simulink model "controladorNovo2015"  (R2018a)
settings: Solver=VariableStepAuto  StartTime=0.0  StopTime=Tsimu  FixedStep=h  RelTol=1e-3
values from neighbouring files (symbols this model uses):
  G = [1; 1]    [init.m]
  h = 0.01    [init.m]
  P0 = eye(2)*1e-4*100    [init.m]
  Qn = 0.01    [init.m]
  R = 0.01    [init.m]
  x0 = x0barra + epsilon    [init.m]
  x0hat = x0barra    [init.m]
undefined symbols (not defined in the file or in its folder): C, Cd, gama, H, phi, Tsimu
libraries: dspinverses x2, dspsrcs4 x1
settings Model: Creator=Raposo  LastModifiedBy=Raposo
settings OptimizationCC: LifeSpan=inf
settings DebuggingCC: AllowSymbolicDim=off  SFExecutionAtInitializationDiag=none
settings HardwareCC: ProdBitPerSizeT=32  ProdBitPerPtrDiffT=32  ProdWordSize=32  ProdHWDeviceType=Specified
settings CodeAppCC: StateflowObjectComments=on

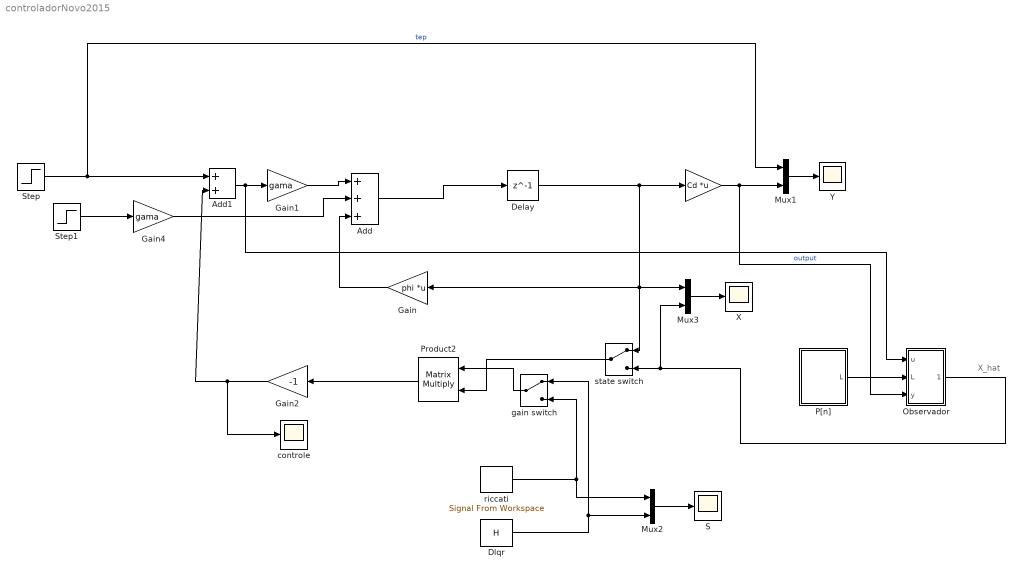
== system controladorNovo2015 ==
  note: X_hat
  " " : Gain  Gain=Cd  Multiplication=Matrix(K*u)
  Add : Sum  Inputs=+++
  Add1 : Sum
  Delay : Delay  DelayLength=1  InitialCondition=x0  SampleTime=h
  Dlqr : Constant  Value=H  VectorParams1D=off
  Gain : Gain  Gain=phi  Multiplication=Matrix(K*u)
  Gain1 : Gain  Gain=gama
  Gain2 : Gain  Gain=-1
  Gain4 : Gain  Gain=gama
  Mux1 : Mux  Inputs=2
  Mux2 : Mux  Inputs=2
  Mux3 : Mux  Inputs=2
  "Observador " : Subsystem
  P[n] : Subsystem
  Product2 : Product  Multiplication=Matrix(*)
  S : Scope
  Step : Step  Time=Tsimu/2  SampleTime=h
  Step1 : Step  Time=10  After=0  SampleTime=1
  X : Scope
  Y : Scope
  controle : Scope
  gain switch : ManualSwitch
  riccati : dspsrcs4/Signal From Workspace  X=lx'  Ts=1  nsamps=1  OutputAfterFinalValue=Setting to zero  ignoreOrWarnInputAndFrameLengths=off  OutputFrames=on
  state switch : ManualSwitch
  wires:
  Gain/1 -> Add/3
  Delay/1 -> Mux3/1, state switch/1, Gain/1, " "/1
  riccati/1 -> Mux2/1, gain switch/2
  Step/1 -> Mux1/1, Add1/1  "tep"
  Mux1/1 -> Y/1
  " "/1 -> "Observador "/3("y "), Mux1/2  "output"
  Mux2/1 -> S/1
  Add1/1 -> "Observador "/1(u), Gain1/1
  Gain1/1 -> Add/1
  Add/1 -> Delay/1
  Product2/1 -> Gain2/1
  Gain2/1 -> controle/1, Add1/2
  Dlqr/1 -> Mux2/2, gain switch/1
  gain switch/1 -> Product2/1
  P[n]/1(L) -> "Observador "/2(L)
  state switch/1 -> Product2/2
  "Observador "/1(Out1) -> Mux3/2, state switch/2
  Mux3/1 -> X/1
  Gain4/1 -> Add/2
  Step1/1 -> Gain4/1

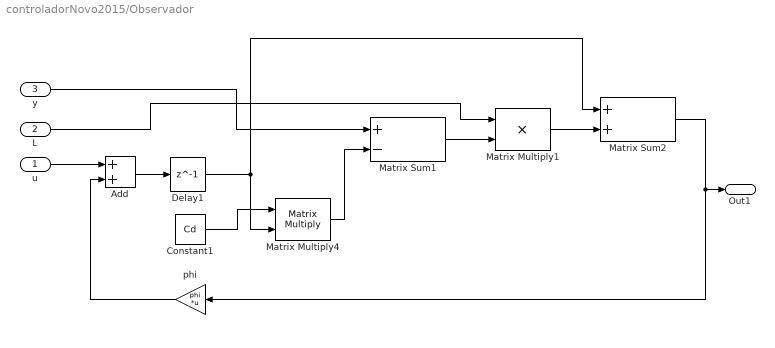
== system controladorNovo2015/Observador  ==
  u : Inport
  L : Inport  Port=2
  "y " : Inport  Port=3
  Add : Sum
  Constant1 : Constant  Value=Cd  VectorParams1D=off
  Delay1 : Delay  DelayLength=1  InitialCondition=x0hat
  Matrix Sum1 : Sum  Inputs=+-
  Matrix Sum2 : Sum
  Matrix Multiply1 : Product  Inputs=**
  Matrix Multiply4 : Product  Inputs=**  Multiplication=Matrix(*)
  phi : Gain  Gain=phi  Multiplication=Matrix(K*u)
  Out1 : Outport
  wires:
  phi/1 -> Add/2
  u/1 -> Add/1
  Add/1 -> Delay1/1
  Matrix Sum2/1 -> Out1/1, phi/1
  "y "/1 -> Matrix Sum1/1
  Delay1/1 -> Matrix Multiply4/2, Matrix Sum2/1
  L/1 -> Matrix Multiply1/1
  Constant1/1 -> Matrix Multiply4/1
  Matrix Multiply4/1 -> Matrix Sum1/2
  Matrix Sum1/1 -> Matrix Multiply1/2
  Matrix Multiply1/1 -> Matrix Sum2/2

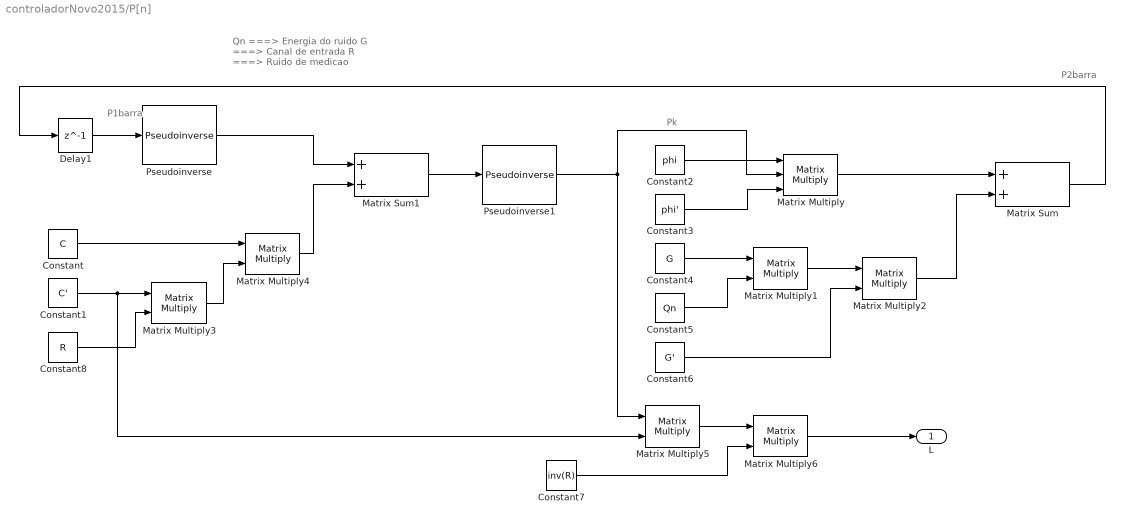
== system controladorNovo2015/P[n] ==
  note: Pk
  note: Qn ===> Energia do ruido
      | G   ===> Canal de entrada
      | R   ===> Ruido de medicao
  note: P2barra
  note: P1barra
  Constant : Constant  Value=C  VectorParams1D=off
  Constant1 : Constant  Value=C'  VectorParams1D=off
  Constant2 : Constant  Value=phi  VectorParams1D=off
  Constant3 : Constant  Value=phi'  VectorParams1D=off
  Constant4 : Constant  Value=G  VectorParams1D=off
  Constant5 : Constant  Value=Qn  VectorParams1D=off
  Constant6 : Constant  Value=G'  VectorParams1D=off
  Constant7 : Constant  Value=inv(R)  VectorParams1D=off
  Constant8 : Constant  Value=R  VectorParams1D=off
  Delay1 : Delay  DelayLength=1  InitialCondition=P0
  Matrix Sum : Sum
  Matrix Sum1 : Sum
  Matrix Multiply : Product  Inputs=***  Multiplication=Matrix(*)
  Matrix Multiply{1..6} (6 alike) : Product  Inputs=**  Multiplication=Matrix(*)
  Pseudoinverse : dspinverses/Pseudoinverse  wanterr=off  SimulateUsing=Interpreted execution
      settings: SourceProductName=DSP System Toolbox  SourceProductBaseCode=DS
  Pseudoinverse1 : dspinverses/Pseudoinverse  wanterr=off  SimulateUsing=Interpreted execution
      settings: SourceProductName=DSP System Toolbox  SourceProductBaseCode=DS
  L : Outport
  wires:
  Pseudoinverse1/1 -> Matrix Multiply5/1, Matrix Multiply/2
  Matrix Sum/1 -> Delay1/1
  Matrix Multiply6/1 -> L/1
  Delay1/1 -> Pseudoinverse/1
  Constant/1 -> Matrix Multiply4/1
  Constant1/1 -> Matrix Multiply5/2, Matrix Multiply3/1
  Constant2/1 -> Matrix Multiply/1
  Constant3/1 -> Matrix Multiply/3
  Constant4/1 -> Matrix Multiply1/1
  Constant5/1 -> Matrix Multiply1/2
  Constant6/1 -> Matrix Multiply2/2
  Matrix Multiply/1 -> Matrix Sum/1
  Matrix Multiply1/1 -> Matrix Multiply2/1
  Matrix Multiply2/1 -> Matrix Sum/2
  Constant8/1 -> Matrix Multiply3/2
  Matrix Multiply3/1 -> Matrix Multiply4/2
  Matrix Multiply4/1 -> Matrix Sum1/2
  Pseudoinverse/1 -> Matrix Sum1/1
  Matrix Sum1/1 -> Pseudoinverse1/1
  Matrix Multiply5/1 -> Matrix Multiply6/1
  Constant7/1 -> Matrix Multiply6/2
